simulink model "heater_autoff"  (R2016a)
settings: Solver=FixedStepDiscrete  StartTime=0.0  StopTime=10.0  RelTol=1e-3
libraries: simulink x1
settings Model: Creator=Stephen  LastModifiedBy=curtm

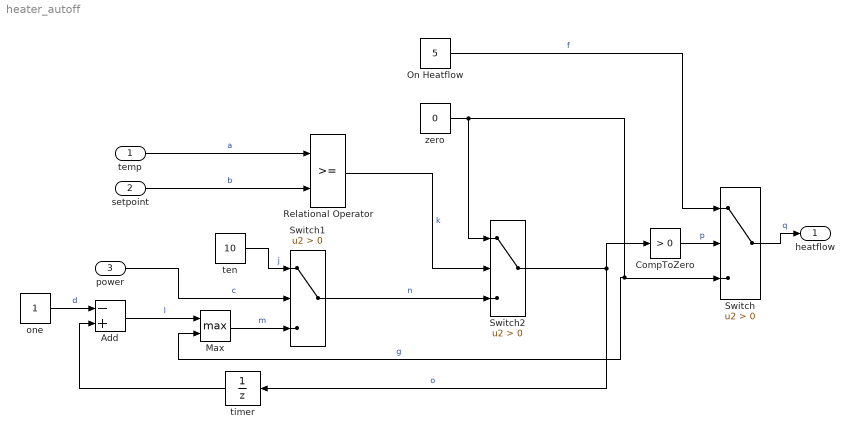
== system heater_autoff ==
  temp : Inport  OutDataTypeStr=double  PortDimensions=1
  setpoint : Inport  Port=2  OutDataTypeStr=double  PortDimensions=1
  power : Inport  Port=3  OutDataTypeStr=boolean  PortDimensions=1
  Add : Sum  Inputs=-+
  CompToZero : simulink/Logic and Bit Operations/Compare To Zero  relop=>  OutDataTypeStr=boolean
  Max : MinMax  Function=max  Inputs=2
  On Heatflow : Constant  Value=5
  Relational Operator : RelationalOperator  OutDataTypeStr=boolean
  Switch : Switch  Criteria=u2 > Threshold
  Switch1 : Switch  Criteria=u2 > Threshold
  Switch2 : Switch  Criteria=u2 > Threshold
  one : Constant
  ten : Constant  Value=10
  timer : UnitDelay  SampleTime=-1
  zero : Constant  Value=0
  heatflow : Outport
  wires:
  power/1 -> Switch1/2  "c"
  temp/1 -> Relational Operator/1  "a"
  CompToZero/1 -> Switch/2  "p"
  setpoint/1 -> Relational Operator/2  "b"
  Switch/1 -> heatflow/1  "q"
  ten/1 -> Switch1/1  "j"
  one/1 -> Add/1  "d"
  Switch2/1 -> timer/1, CompToZero/1  "o"
  On Heatflow/1 -> Switch/1  "f"
  zero/1 -> Max/2, Switch/3, Switch2/1  "g"
  Max/1 -> Switch1/3  "m"
  Add/1 -> Max/1  "l"
  Relational Operator/1 -> Switch2/2  "k"
  Switch1/1 -> Switch2/3  "n"
  timer/1 -> Add/2
